simulink model "testeCAFaseA"  (R2015a)
settings: Solver=FixedStepDiscrete  StartTime=0.0  StopTime=4.5  RelTol=1e-3
PreLoadFcn:
  | Ts=20e-6;
undefined symbols (not defined in the file or in its folder): driveGuiManager, gcbh, sps_rtmsupport
libraries: powerlib x20, powerlib_meascontrol x17, simulink_extras x3, spsDrivesOutputSelector x1
(part 2 of 2)

== system testeCAFaseA/Six-Step VSI Induction Motor Drive/Bridge firing unit/Discrete Synchronized 6-Pulse Generator/6 Flip-Flop/S-R Flip-Flop5 ==
  S : Inport
  R : Inport  Port=2
  Demux : Demux  Outputs=2
  Logic : CombinatorialLogic  TruthTable=[0 1;0 1;1 0;0 1;1 0;0 1;1 0;1 0]
  Mux : Mux  Inputs=3
  Unit Delay : UnitDelay  InitialCondition=initial_condition  SampleTime=Ts
  Q : Outport  InitialOutput=0
  !Q : Outport  Port=2  InitialOutput=1
  wires:
  Mux/1 -> Logic/1
  Logic/1 -> Demux/1
  Demux/2 -> !Q/1
  Demux/1 -> Q/1, Unit Delay/1
  Unit Delay/1 -> Mux/1
  S/1 -> Mux/2
  R/1 -> Mux/3

== system testeCAFaseA/Six-Step VSI Induction Motor Drive/Bridge firing unit/Discrete Synchronized 6-Pulse Generator/6 Flip-Flop/S-R Flip-Flop6 ==
  S : Inport
  R : Inport  Port=2
  Demux : Demux  Outputs=2
  Logic : CombinatorialLogic  TruthTable=[0 1;0 1;1 0;0 1;1 0;0 1;1 0;1 0]
  Mux : Mux  Inputs=3
  Unit Delay : UnitDelay  InitialCondition=initial_condition  SampleTime=Ts
  Q : Outport  InitialOutput=0
  !Q : Outport  Port=2  InitialOutput=1
  wires:
  R/1 -> Mux/3
  S/1 -> Mux/2
  Unit Delay/1 -> Mux/1
  Demux/1 -> Unit Delay/1, Q/1
  Demux/2 -> !Q/1
  Logic/1 -> Demux/1
  Mux/1 -> Logic/1
